simulink model "FNM_00_Colocar_em_Condicoes_Iniciais"  (Simulink 7.1)
settings: Solver=ode45  StartTime=0.0  StopTime=3000  RelTol=1e-3
undefined symbols (not defined in the file or in its folder): analoginput, analogoutput, QT
libraries: simulink x3, daqlib x2
settings Model: Creator=didaticontrol  LastModifiedBy=didaticontrol

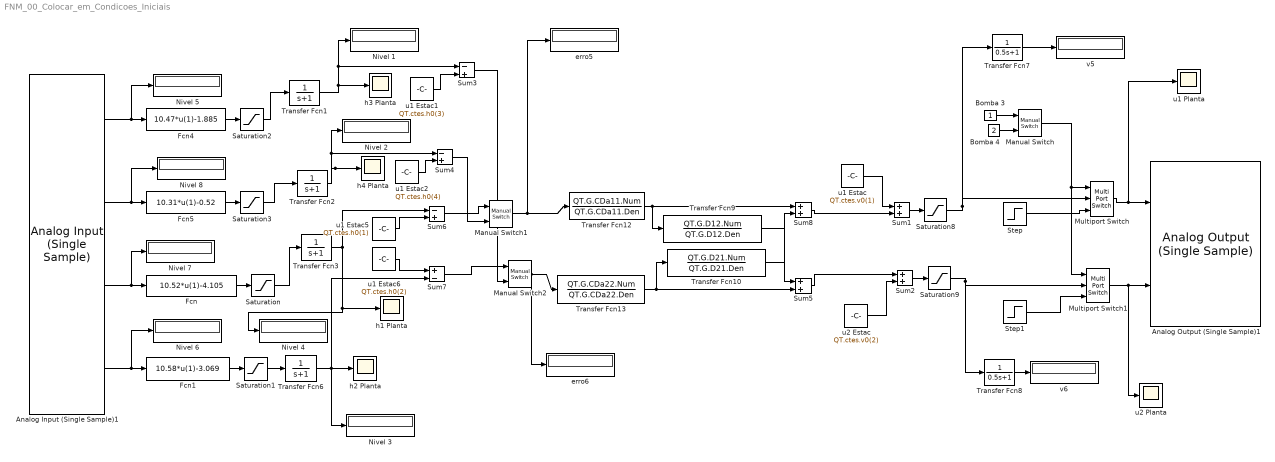
== system FNM_00_Colocar_em_Condicoes_Iniciais ==
  Analog Input (Single Sample)1 : daqlib/Analog Input (Single Sample)  DialogController=daqcreatedialog  DialogControllerArgs=DataTag0  DeviceMenu=nidaq Dev1 (USB-6008)  Device=nidaq Dev1 (USB-6008)  ObjConstructor=analoginput('nidaq','Dev1')  InputType=Differential  NChannelsSelected=4  Channels=1$0$$2$#1$1$$2$#1$2$$2$#1$3$$2$#  NPorts=1 per hardware channel  BlockSampleTime=10e-3
  Analog Output (Single Sample)1 : daqlib/Analog Output (Single Sample)  DialogController=daqcreatedialog  DialogControllerArgs=DataTag1  DeviceMenu=nidaq Dev1 (USB-6008)  Device=nidaq Dev1 (USB-6008)  ObjConstructor=analogoutput('nidaq','Dev1')  NChannelsSelected=2  Channels=1$0$$1$0$#1$1$$1$0$#  NPorts=1 per hardware channel
  Bomba 3 : Constant
  Bomba 4 : Constant  Value=2
  Fcn : Fcn  Expr=10.52*u(1)-4.105  SampleTime=10e-3
  Fcn1 : Fcn  Expr=10.58*u(1)-3.069
  Fcn4 : Fcn  Expr=10.47*u(1)-1.885
  Fcn5 : Fcn  Expr=10.31*u(1)-0.52
  Manual Switch : simulink/Signal Routing/Manual Switch  SystemSampleTime=-1  sw=0  action=0  varsize=off
  Manual Switch1 : simulink/Signal Routing/Manual Switch  SystemSampleTime=-1  sw=1  action=0  varsize=off
  Manual Switch2 : simulink/Signal Routing/Manual Switch  SystemSampleTime=-1  sw=1  action=0  varsize=off
  Multiport Switch : MultiPortSwitch  Inputs=2  OutDataType=sfix(16)  OutScaling=2^0
  Multiport Switch1 : MultiPortSwitch  Inputs=2  OutDataType=sfix(16)  OutScaling=2^0
  Nivel {1..8} (8 alike) : Display
  Saturation : Saturate  UpperLimit=23  LowerLimit=0  SampleTime=10e-3
  Saturation1 : Saturate  UpperLimit=23  LowerLimit=0
  Saturation2 : Saturate  UpperLimit=23  LowerLimit=0
  Saturation3 : Saturate  UpperLimit=23  LowerLimit=0
  Saturation8 : Saturate  UpperLimit=0.7*5  LowerLimit=0  SampleTime=10e-3
  Saturation9 : Saturate  UpperLimit=0.7*5  LowerLimit=0  SampleTime=10e-3
  Step : Step  Time=70  Before=QT.ctes.v0(1)  After=QT.ctes.v0(1)+0.15
  Step1 : Step  Time=450  Before=QT.ctes.v0(2)  After=QT.ctes.v0(2)+0.15
  Sum{1..2,5,8} (4 alike) : Sum  OutDataType=sfix(16)  OutScaling=2^0
  Sum3 : Sum  Inputs=-+  OutDataType=sfix(16)  OutScaling=2^0
  Sum4 : Sum  Inputs=-+  OutDataType=sfix(16)  OutScaling=2^0
  Sum6 : Sum  Inputs=-+  OutDataType=sfix(16)  OutScaling=2^0
  Sum7 : Sum  Inputs=+-  OutDataType=sfix(16)  OutScaling=2^0
  Transfer Fcn{1..3,6} (4 alike) : TransferFcn  Denominator=[1 1]
  Transfer Fcn10 : TransferFcn  Numerator=QT.G.D21.Num  Denominator=QT.G.D21.Den
  Transfer Fcn12 : TransferFcn  Numerator=QT.G.CDa11.Num  Denominator=QT.G.CDa11.Den
  Transfer Fcn13 : TransferFcn  Numerator=QT.G.CDa22.Num  Denominator=QT.G.CDa22.Den
  Transfer Fcn7 : TransferFcn  Denominator=[0.5 1]
  Transfer Fcn8 : TransferFcn  Denominator=[0.5 1]
  Transfer Fcn9 : TransferFcn  Numerator=QT.G.D12.Num  Denominator=QT.G.D12.Den
  erro5 : Display
  erro6 : Display
  h1 Planta : Scope
      settings: TimeRange=500  YMin=0  YMax=8  SaveName=h1_real  SampleInput=on  SampleTime=10e-3
  h2 Planta : Scope
      settings: YMin=0  YMax=8  SaveName=h2_real  SampleInput=on  SampleTime=10e-3
  h3 Planta : Scope
      settings: YMin=0  YMax=8.5  SaveName=h3_real  SampleInput=on  SampleTime=10e-3
  h4 Planta : Scope
      settings: YMin=0  YMax=12  SaveName=h4_real  SampleInput=on  SampleTime=10e-3
  u1 Planta : Scope
      settings: YMin=1.2  YMax=3.5  SaveName=u1_real  SampleInput=on  SampleTime=10e-3
  u1 Estac : Constant  Value=QT.ctes.v0(1)
  u1 Estac1 : Constant  Value=QT.ctes.h0(3)
  u1 Estac2 : Constant  Value=QT.ctes.h0(4)
  u1 Estac5 : Constant  Value=QT.ctes.h0(1)
  u1 Estac6 : Constant  Value=QT.ctes.h0(2)
  u2 Planta : Scope
      settings: YMin=1.7  YMax=3.5  SaveName=u2_real  SampleInput=on  SampleTime=10e-3
  u2 Estac : Constant  Value=QT.ctes.v0(2)
  v5 : Display
  v6 : Display
  wires:
  Analog Input (Single Sample)1/3 -> Fcn/1, Nivel 7/1
  Fcn/1 -> Saturation/1
  Fcn1/1 -> Saturation1/1
  Analog Input (Single Sample)1/4 -> Fcn1/1, Nivel 6/1
  Analog Input (Single Sample)1/2 -> Fcn5/1, Nivel 8/1
  Analog Input (Single Sample)1/1 -> Nivel 5/1, Fcn4/1
  Fcn4/1 -> Saturation2/1
  Fcn5/1 -> Saturation3/1
  Multiport Switch1/1 -> Analog Output (Single Sample)1/2, u2 Planta/1
  Sum6/1 -> Manual Switch1/1
  Saturation9/1 -> Transfer Fcn8/1, Multiport Switch1/2
  u1 Estac5/1 -> Sum6/2
  u1 Estac6/1 -> Sum7/1
  Sum1/1 -> Saturation8/1
  u1 Estac/1 -> Sum1/1
  Sum2/1 -> Saturation9/1
  u2 Estac/1 -> Sum2/2
  Multiport Switch/1 -> u1 Planta/1, Analog Output (Single Sample)1/1
  Saturation8/1 -> Transfer Fcn7/1, Multiport Switch/2
  Transfer Fcn1/1 -> h3 Planta/1, Nivel 1/1, Sum3/1
  Saturation2/1 -> Transfer Fcn1/1
  Transfer Fcn2/1 -> h4 Planta/1, Nivel 2/1, Sum4/1
  Saturation3/1 -> Transfer Fcn2/1
  Transfer Fcn3/1 -> Nivel 4/1, h1 Planta/1, Sum6/1
  Saturation/1 -> Transfer Fcn3/1
  Transfer Fcn6/1 -> h2 Planta/1, Nivel 3/1, Sum7/2
  Saturation1/1 -> Transfer Fcn6/1
  Transfer Fcn7/1 -> v5/1
  Transfer Fcn8/1 -> v6/1
  Manual Switch/1 -> Multiport Switch/1, Multiport Switch1/1
  Step1/1 -> Multiport Switch1/3
  Bomba 3/1 -> Manual Switch/1
  Bomba 4/1 -> Manual Switch/2
  u1 Estac1/1 -> Sum3/2
  Sum3/1 -> Manual Switch2/2
  u1 Estac2/1 -> Sum4/2
  Manual Switch1/1 -> erro5/1, Transfer Fcn12/1
  Sum4/1 -> Manual Switch1/2
  Manual Switch2/1 -> erro6/1, Transfer Fcn13/1
  Sum7/1 -> Manual Switch2/1
  Transfer Fcn12/1 -> Transfer Fcn9/1, Sum8/1
  Transfer Fcn13/1 -> Transfer Fcn10/1, Sum5/2
  Sum8/1 -> Sum1/2
  Transfer Fcn10/1 -> Sum8/2
  Sum5/1 -> Sum2/1
  Transfer Fcn9/1 -> Sum5/1
  Step/1 -> Multiport Switch/3
